simulink model "twolink_PD_sliding_soft"  (R2022b)
settings: Solver=FixedStepAuto  StartTime=0.0  StopTime=t_max  FixedStep=dt_max  RelTol=1e-3
values from neighbouring files (symbols this model uses):
  h = 1/delta^(alpha/beta)    (= 16)    [smc.m]
  k = 5    [smc.m]
  K1 = ones(n,1)*20    [smc.m]
  K2 = ones(n,1)*2    [smc.m]
  l = 7    [smc.m]
  m = 3    [mpc_script.m]    (also in smc.m = 7)
  mu_1 = 1    [smc.m]
  mu_2 = 3    [smc.m]
  p = 10    [mpc_script.m]    (also in smc.m = 5)
  phi = 0.2    [smc.m]
  theta_0 = zeros(n,1)    [mpc_script.m]    (also in smc.m)
  theta_dot0 = zeros(n,1)    [mpc_script.m]    (also in smc.m)
libraries: simulink x3
settings Model: LastModifiedBy=dimitriasilveria
settings OptimizationCC: BlockReduction=off  BooleanDataType=off
settings DebuggingCC: SaveWithParameterizedLinksMsg=none  UnderspecifiedInitializationDetection=Classic  MergeDetectMultiDrivingBlocksExec=none  SignalResolutionControl=TryResolveAllWithWarning
settings HardwareCC: TargetUnknown=on
settings ModelReferenceCC: PropagateSignalLabelsOutOfModel=off

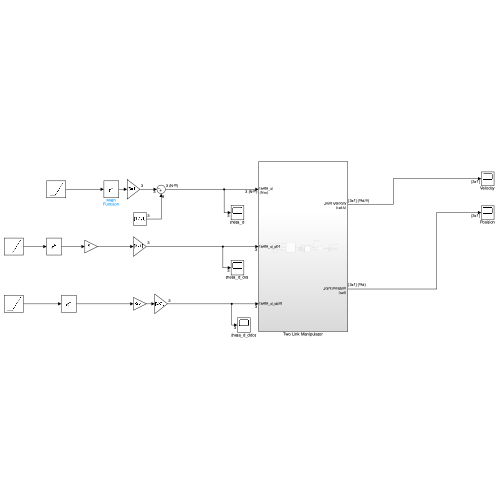
[thumbnail: Simulink's stored preview of the top-level diagram]
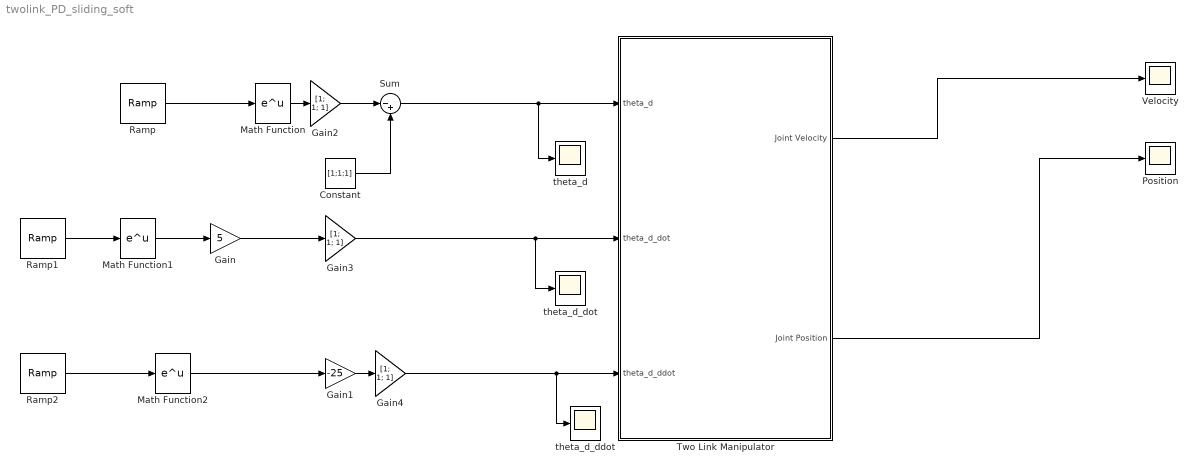
== system twolink_PD_sliding_soft ==
  Constant : Constant  Value=[1;1;1]
  Gain : Gain  Gain=5
  Gain1 : Gain  Gain=-25
  Gain2 : Gain  Gain=[1; 1; 1]
  Gain3 : Gain  Gain=[1; 1; 1]
  Gain4 : Gain  Gain=[1; 1; 1]
  Math Function : Math
  Math Function1 : Math
  Math Function2 : Math
  Position : Scope
  Ramp : simulink/Sources/Ramp  slope=-5  start=0  InitialOutput=0
  Ramp1 : simulink/Sources/Ramp  slope=-5  start=0  InitialOutput=0
  Ramp2 : simulink/Sources/Ramp  slope=-5  start=0  InitialOutput=0
  Sum : Sum  Inputs=|-+
  Two Link Manipulator : Subsystem
  Velocity : Scope
  theta_d : Scope
  theta_d_ddot : Scope
  theta_d_dot : Scope
  wires:
  Two Link Manipulator/1(Joint Velocity) -> Velocity/1
  Two Link Manipulator/2(Joint Position) -> Position/1
  Gain/1 -> Gain3/1
  Gain1/1 -> Gain4/1
  Ramp/1 -> Math Function/1
  Math Function/1 -> Gain2/1
  Constant/1 -> Sum/2
  Sum/1 -> theta_d/1, Two Link Manipulator/1(theta_d)
  Math Function1/1 -> Gain/1
  Ramp1/1 -> Math Function1/1
  Math Function2/1 -> Gain1/1
  Ramp2/1 -> Math Function2/1
  Gain2/1 -> Sum/1
  Gain3/1 -> theta_d_dot/1, Two Link Manipulator/2(theta_d_dot)
  Gain4/1 -> theta_d_ddot/1, Two Link Manipulator/3(theta_d_ddot)

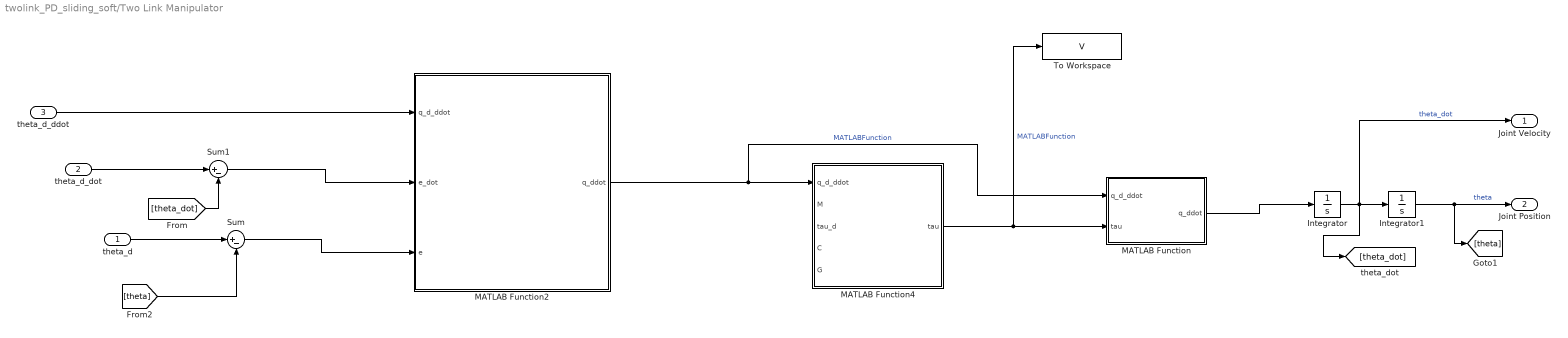
== system twolink_PD_sliding_soft/Two Link Manipulator ==
  theta_d : Inport  Unit=N*m
  theta_d_dot : Inport  Port=2
  theta_d_ddot : Inport  Port=3
  Integrator : Integrator  InitialCondition=theta_dot0
  Integrator1 : Integrator  InitialCondition=theta_0
  MATLAB Function : MATLAB Function  TreatAsAtomicUnit=on
  MATLAB Function2 : MATLAB Function  TreatAsAtomicUnit=on
  MATLAB Function4 : MATLAB Function  TreatAsAtomicUnit=on
  Sum : Sum  Inputs=|+-
  Sum1 : Sum  Inputs=|+-
  To Workspace : ToWorkspace  VariableName=V  SaveFormat=Timeseries  SampleTime=-1
  Joint Velocity : Outport  Unit=rad/s
  Joint Position : Outport  Port=2  Unit=rad
  wires:
  Integrator/1 -> [theta_dot], Joint Velocity/1, Integrator1/1  "theta_dot"
  Integrator1/1 -> [theta], Joint Position/1  "theta"
  theta_d/1 -> Sum/1
  MATLAB Function2/1(q_ddot) -> MATLAB Function/1(q_d_ddot), MATLAB Function4/1(q_d_ddot)  "MATLABFunction"
  [theta] -> Sum/2
  MATLAB Function4/1(tau) -> To Workspace/1, MATLAB Function/2(tau)  "MATLABFunction"
  theta_d_dot/1 -> Sum1/1
  [theta_dot] -> Sum1/2
  Sum/1 -> MATLAB Function2/3(e)
  Sum1/1 -> MATLAB Function2/2(e_dot)
  theta_d_ddot/1 -> MATLAB Function2/1(q_d_ddot)
  MATLAB Function/1(q_ddot) -> Integrator/1

== matlab function twolink_PD_sliding_soft/Two Link Manipulator/MATLAB Function ==
  data: q_d_ddot input; tau input; q_ddot output
function q_ddot = dynamics(q_d_ddot,tau)
q_ddot = q_d_ddot;

%dynamics here

== matlab function twolink_PD_sliding_soft/Two Link Manipulator/MATLAB Function2 ==
  data: q_d_ddot input; e_dot input; q_ddot output; p parameter; k parameter; m parameter; l parameter; K1 parameter; K2 parameter; h parameter; phi parameter; e input; mu_2 parameter; mu_1 parameter
function q_ddot  = sliding_surface_to_acceleration(q_d_ddot,e_dot,p, k, m, l, K1, K2, h, phi, e, mu_2, mu_1)
s =e_dot + mu_1*e.^(m/p)+mu_2*e.^(k/l);
if abs(s)>=phi
    sat = sign(s);
else
    sat=h*s;
end
s_dot = -K1.*s-K2.*sat;

q_ddot = q_d_ddot + mu_1*(m/p)*e.^((m/p)-1).*e_dot + mu_2*(k/l)*e.^((k/l)-1).*e_dot - s_dot;

== matlab function twolink_PD_sliding_soft/Two Link Manipulator/MATLAB Function4 ==
  data: q_d_ddot input; M input; tau output; tau_d input; C input; G input; n parameter
function tau = inpute_torque(q_d_ddot,M,tau_d, C, G,n)
%here I am assuming C = C(q,q_dot)*q_dot,

tau = M*q_d_ddot + C + G -tau_d;
